simulink model "task_3e"  (R2014b)
settings: Solver=ode45  StartTime=0.0  StopTime=450  RelTol=1e-3
values from neighbouring files (symbols this model uses):
  A = [-0.322 0.052 0.028 -1.12 ... (first row only)    [parameters.m]
  B = [0.002 0 -0.65 -0.02]'    [parameters.m]
  C = [0 0 0 1 ... (first row only)    [parameters.m]
  E = eye(4)    [parameters.m]
  g = 9.81    [parameters.m]
  Kd_phi = 2.15    [parameters.m]
  Ki_chi = 0.1954    [parameters.m]
  Kp_chi = 3.7547    [parameters.m]
  Kp_phi = -5/3    (= -1.66666666667)    [parameters.m]
  P0 = zeros(4,4)    [parameters.m]
  p_noisePower = (0.5/180)^2    (= 7.71604938272e-06)    [parameters.m]
  phi_noisePower = (2/180)^2    (= 0.000123456790123)    [parameters.m]
  Q = diag(Q)    [parameters.m]
  R_inv = inv(R)    [parameters.m]
  r_noisePower = (0.2/180)^2    (= 1.23456790123e-06)    [parameters.m]
  Vg = 637/3.6    (= 176.944444444)    [parameters.m]
libraries: simulink x3
settings Model: Creator=sondr_000  LastModifiedBy=Ultrawack
settings OptimizationCC: BlockReduction=off  BooleanDataType=off  UseDivisionForNetSlopeComputation=off  SimCompilerOptimization=off
settings DebuggingCC: SaveWithParameterizedLinksMsg=none  UnderspecifiedInitializationDetection=Classic  MergeDetectMultiDrivingBlocksExec=none  SignalResolutionControl=TryResolveAllWithWarning  SolverPrmCheckMsg=none  FcnCallInpInsideContextMsg=error  FrameProcessingCompatibilityMsg=error  SFExecutionAtInitializationDiag=none
settings HardwareCC: ProdBitPerSizeT=32  ProdBitPerPtrDiffT=32  TargetUnknown=on
settings RTWCC: RTWCompilerOptimization=off
settings ConfigComp: CovMetricSettings=dw  CovHtmlReporting=on  CovSaveCumulativeToWorkspaceVar=on  CovSaveSingleToWorkspaceVar=on  CovExternalEMLEnable=off  CovSFcnEnable=off

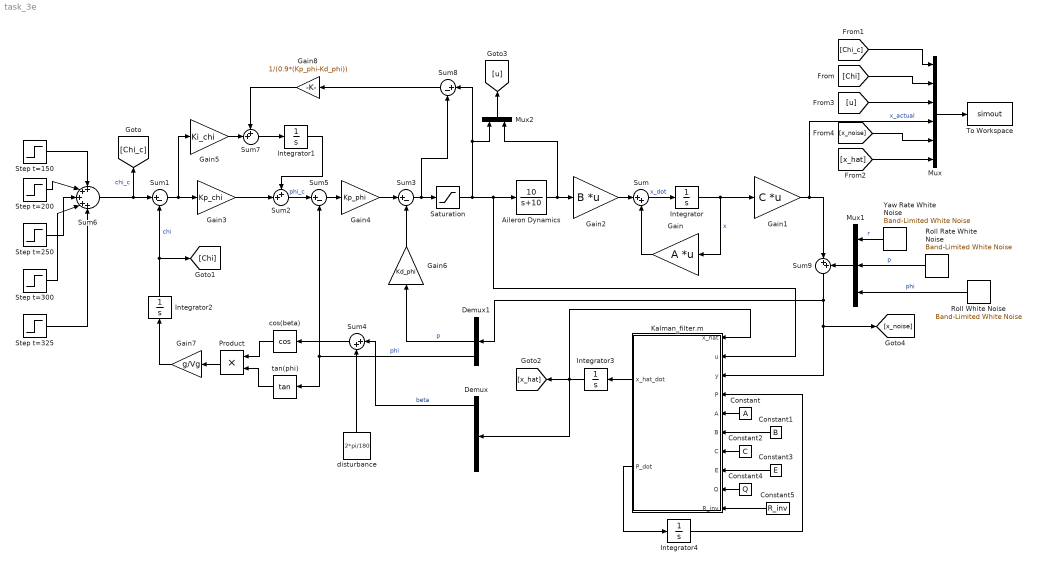
== system task_3e ==
  Aileron Dynamics : TransferFcn  Numerator=[10]  Denominator=[1 10]
  Constant : Constant  Value=A
  Constant1 : Constant  Value=B
  Constant2 : Constant  Value=C
  Constant3 : Constant  Value=E
  Constant4 : Constant  Value=Q
  Constant5 : Constant  Value=R_inv
  Demux : Demux
  Demux1 : Demux  Outputs=3
  Gain : Gain  Gain=A  Multiplication=Matrix(K*u)
  Gain1 : Gain  Gain=C  Multiplication=Matrix(K*u)
  Gain2 : Gain  Gain=B  Multiplication=Matrix(K*u)
  Gain3 : Gain  Gain=Kp_chi
  Gain4 : Gain  Gain=Kp_phi
  Gain5 : Gain  Gain=Ki_chi
  Gain6 : Gain  Gain=Kd_phi
  Gain7 : Gain  Gain=g/Vg
  Gain8 : Gain  Gain=1/(0.9*(Kp_phi-Kd_phi))
  Integrator : Integrator
  Integrator1 : Integrator
  Integrator2 : Integrator
  Integrator3 : Integrator  InitialCondition=[0 0 0 0]
  Integrator4 : Integrator  InitialCondition=P0
  Kalman_filter.m : MATLAB Function  TreatAsAtomicUnit=on
  Mux : Mux  Inputs=6
  Mux1 : Mux  Inputs=3
  Mux2 : Mux  Inputs=2
  Product : Product
  Roll White Noise : simulink/Sources/Band-Limited White Noise  Cov=[phi_noisePower]  Ts=0.1  seed=[95125]
  Roll Rate White Noise : simulink/Sources/Band-Limited White Noise  Cov=[p_noisePower]  Ts=0.1  seed=[54201]
  Saturation : Saturate  UpperLimit=25*pi/180  LowerLimit=-025*pi/180
  Step t=150 : Step  Time=100  After=0.20  SampleTime=0
  Step t=200 : Step  Time=200  After=0.15  SampleTime=0
  Step t=250 : Step  Time=220  After=0.20  SampleTime=0
  Step t=300 : Step  Time=300  After=0.25  SampleTime=0
  Step t=325 : Step  Time=375  After=-0.10  SampleTime=0
  Sum : Sum  Inputs=|++
  Sum{1,3,5,8} (4 alike) : Sum  Inputs=|+-
  Sum2 : Sum  Inputs=++|
  Sum4 : Sum  Inputs=|++
  Sum6 : Sum  Inputs=+++++
  Sum7 : Sum  Inputs=++|
  Sum9 : Sum  Inputs=|++
  To Workspace : ToWorkspace  VariableName=simout  SaveFormat=Timeseries  SampleTime=-1
  Yaw Rate White Noise : simulink/Sources/Band-Limited White Noise  Cov=[r_noisePower]  Ts=0.1  seed=[23341]
  cos(beta) : Trigonometry  Operator=cos
  disturbance : Constant  Value=2*pi/180
  tan(phi) : Trigonometry  Operator=tan
  wires:
  Gain1/1 -> Mux/4, Sum9/1  "x_actual"
  Integrator/1 -> Gain1/1, Gain/1  "x"
  Sum/1 -> Integrator/1  "x_dot"
  Gain/1 -> Sum/2
  Gain2/1 -> Sum/1
  Saturation/1 -> Aileron Dynamics/1, Kalman_filter.m/2(u), Mux2/1, Sum8/1
  Sum1/1 -> Gain5/1, Gain3/1
  Sum3/1 -> Sum8/2, Saturation/1
  Gain4/1 -> Sum3/1
  Gain6/1 -> Sum3/2
  Sum6/1 -> Sum1/1, [Chi_c]  "chi_c"
  Gain3/1 -> Sum2/2
  Sum5/1 -> Gain4/1
  Sum2/1 -> Sum5/1  "phi_c"
  Mux/1 -> To Workspace/1
  Integrator2/1 -> Sum1/2, [Chi]  "chi"
  Gain7/1 -> Integrator2/1
  tan(phi)/1 -> Product/2
  cos(beta)/1 -> Product/1
  Product/1 -> Gain7/1
  Sum4/1 -> cos(beta)/1
  disturbance/1 -> Sum4/2
  Step t=150/1 -> Sum6/1
  Step t=200/1 -> Sum6/2
  Step t=250/1 -> Sum6/3
  Step t=300/1 -> Sum6/4
  Step t=325/1 -> Sum6/5
  Integrator1/1 -> Sum2/1
  Sum7/1 -> Integrator1/1
  Gain5/1 -> Sum7/2
  Sum8/1 -> Gain8/1
  Gain8/1 -> Sum7/1
  Kalman_filter.m/1(x_hat_dot) -> Integrator3/1
  Integrator4/1 -> Kalman_filter.m/4(P)
  Kalman_filter.m/2(P_dot) -> Integrator4/1
  Integrator3/1 -> Demux/1, [x_hat], Kalman_filter.m/1(x_hat)
  Sum9/1 -> Kalman_filter.m/3(y), [x_noise], Demux1/1
  Demux/1 -> Sum4/1  "beta"
  Demux1/3 -> tan(phi)/1, Sum5/2  "phi"
  Demux1/2 -> Gain6/1  "p"
  Mux1/1 -> Sum9/2
  Yaw Rate White Noise/1 -> Mux1/1  "r"
  Roll Rate White Noise/1 -> Mux1/2  "p"
  Roll White Noise/1 -> Mux1/3  "phi"
  Constant/1 -> Kalman_filter.m/5(A)
  Constant1/1 -> Kalman_filter.m/6(B)
  Constant2/1 -> Kalman_filter.m/7(C)
  Constant3/1 -> Kalman_filter.m/8(E)
  Constant4/1 -> Kalman_filter.m/9(Q)
  Constant5/1 -> Kalman_filter.m/10(R_inv)
  [Chi_c] -> Mux/1
  [Chi] -> Mux/2
  [x_hat] -> Mux/6
  [x_noise] -> Mux/5
  [u] -> Mux/3
  Aileron Dynamics/1 -> Gain2/1, Mux2/2
  Mux2/1 -> [u]

== matlab function task_3e/Kalman_filter.m ==
  data: x_hat input; u input; y input; P input; x_hat_dot output; P_dot output; A input; B input; C input; E input; Q input; R_inv input
function [ x_hat_dot, P_dot ] = Kalman_filter( x_hat, u, y, P , A, B, C, E, Q, R_inv)
K = P*C'*R_inv;
x_hat_dot = A*x_hat + B*u + K*(y - C*x_hat);
P_dot = A*P + P*A' + E*Q*E' - P*C'*R_inv*C*P;
end
